simulink model "Ivanov_9_airplane"  (Simulink 10.0)
settings: Solver=FixedStepAuto  StartTime=0.0  StopTime=50.0  RelTol=1e-3
undefined symbols (not defined in the file or in its folder): DiscIntNeverNeededParam
libraries: aerolibanim x1
settings Model: Creator=prime  LastModifiedBy=prime
settings DataIOCC: SaveFormat=Dataset  ReturnWorkspaceOutputs=on
settings OptimizationCC: LifeSpan=auto
settings DebuggingCC: UnderspecifiedInitializationDetection=Simplified  MergeDetectMultiDrivingBlocksExec=error  SFUnexpectedBacktrackingDiag=error  SFNoUnconditionalDefaultTransitionDiag=error  SFExecutionAtInitializationDiag=warning  ArithmeticOperatorsInVariantConditions=error
settings HardwareCC: ProdBitPerPointer=64  ProdBitPerSizeT=64  ProdBitPerPtrDiffT=64  ProdLargestAtomicFloat=Float  ProdIntDivRoundTo=Zero  ProdEndianess=LittleEndian  ProdWordSize=64  ProdHWDeviceType=Intel->x86-64 (Windows64)
settings ModelReferenceCC: PropagateSignalLabelsOutOfModel=on
settings SFSimCC: SimUseLocalCustomCode=on  CustomCodeUndefinedFunction=FilterOut
settings RTWCC: RTWUseLocalCustomCode=on
settings CodeAppCC: StateflowObjectComments=off
settings GRTTargetCC: TargetLangStandard=C99 (ISO)  CombineOutputUpdateFcns=on  GRTInterface=off
settings ConfigComp: CovMetricSettings=dwe  CovHtmlReporting=off  CovSaveCumulativeToWorkspaceVar=off  CovSaveSingleToWorkspaceVar=off

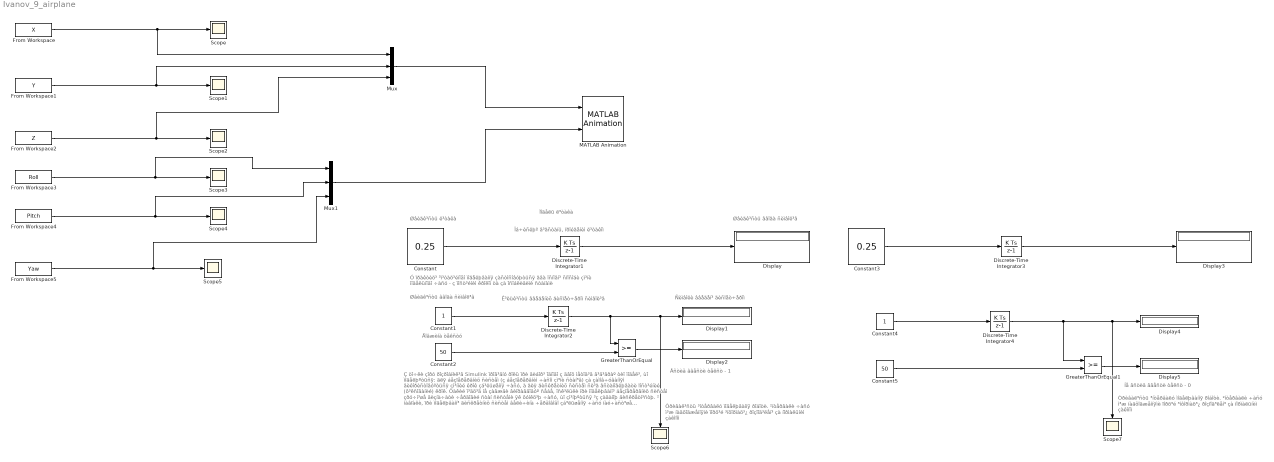
== system Ivanov_9_airplane ==
  note: Ñèìâîëè ââåäåí³ äèñïåò÷åðîì
  note: Øâèäê³ñòü ââîäà ñèìâîë³â
  note: Äîâæèíà òåêñòó
  note: Øâèäê³ñòü ë³òàêà
  note: Øâèäê³ñòü ââîäà ñèìâîë³â
  note: Âñòèã ââåñòè òåêñò - 1
  note: Îá÷èñëþº â³äñòàíü, ïðîéäåíèì ë³òàêîì
  note: Òðèâàë³ñòü ³íòåðâàëó ìîäåëþâàííÿ ðîáîòè.
      | ²íòåðâàëè ÷àñó ì³æ íàäõîäæåííÿìè ïîðö³é ³íôîðìàö³¿ ðîçïîä³ëåí³ çà íîðìàëüíèì çàêîíîì
  note: Íå âñòèã ââåñòè òåêñò - 0
  note: Òðèâàë³ñòü ³íòåðâàëó ìîäåëþâàííÿ ðîáîòè.
      | ²íòåðâàëè ÷àñó ì³æ íàäõîäæåííÿìè ïîðö³é ³íôîðìàö³¿ ðîçïîä³ëåí³ çà íîðìàëüíèì çàêîíîì
  note: Ê³ëüê³ñòü ââåäåíèõ äèñïåò÷åðîì ñèìâîë³â
  note: Ó ïðàêòèö³ ³ì³òàö³éíîãî ìîäåëþâàííÿ çàñòîñîâóþòüñÿ äâà îñíîâí³ ñïîñîáè çì³íè ìîäåëüíîãî ÷àñó - ç ïîñò³éíèì êðîêîì òà çà îñîáëèâèìè ñòàíàìè
  note: Ç òî÷êè çîðó ðîçðîáíèê³â Simulink ïðîâ³äíó ðîëü ïðè âèáîð³ îäíîãî ç äâîõ ìåòîä³â â³ä³ãðàº òèï ìîäåë³, ùî ìîäåëþºòüñÿ: äëÿ áåçïåðåðâíèõ ñèñòåì (ç áåçïåðåðâíèì ÷àñîì çì³íè ñòàí³â) çà çàìîâ÷óâàííÿì âèêîðèñòîâóºòüñÿ çì³ííèé êðîê çá³ëüøåííÿ ÷àñó, à äëÿ äèñêðåòíèõ ñèñòåì ñë³ä âñòàíîâëþâàòè ïîñò³éíèé (ô³êñîâàíèé) êðîê. Òàêèé ï³äõ³ä íå çàâæäè âèïðàâäîâóº ñåáå, îñê³ëüêè ïðè ìîäåëþâàíí³ áåçïåðåðâíèõ ñèñòåì çðó÷í³øå âèçíà÷àòè ÷åðãîâèé ñòàí ñèñòåìè ÿê ôóíêö³þ ÷àñó, ùî çì³íþºòüñÿ ³ç çàäàíîþ äèñêðåòí³ñòþ. ² íàâïàêè, ïðè ìîäåëþâàíí³ äèñêðåòíèõ ñèñòåì âåëè÷èíà ÷åðãîâîãî çá³ëüøåííÿ ÷àñó íàé÷àñò³øå âèçíà÷àºòüñÿ ïðîãíîçîâàíèì ìîìåíòîì çì³íè ñòàíó ñèñòåìè; ïðè÷îìó çì³íà ñòàí³â â³äáóâàºòüñÿ, çàçâè÷àé, íåðåãóëÿðíî. Òîìó êîðèñíî çíàòè, ÿêèì ÷èíîì ðîçðîáêè ìîäåëåé äèñêðåòíèõ ñèñòåì ìîæíà çìóñèòè ìîäåëüíèé ÷àñ çì³íþâàòèñÿ ïî îñîáëèâèì ñòàíàì.
  note: Ìîäåëü ë³òàêà
  Constant : Constant  Value=0.25  SampleTime=2
  Constant1 : Constant  SampleTime=2
  Constant2 : Constant  Value=50  SampleTime=2
  Constant3 : Constant  Value=0.25  SampleTime=3
  Constant4 : Constant  SampleTime=3
  Constant5 : Constant  Value=50  SampleTime=3
  Discrete-Time Integrator1 : DiscreteIntegrator  SampleTime=2  ICPrevOutput=DiscIntNeverNeededParam  ICPrevScaledInput=DiscIntNeverNeededParam
  Discrete-Time Integrator2 : DiscreteIntegrator  SampleTime=2  ICPrevOutput=DiscIntNeverNeededParam  ICPrevScaledInput=DiscIntNeverNeededParam
  Discrete-Time Integrator3 : DiscreteIntegrator  SampleTime=3  ICPrevOutput=DiscIntNeverNeededParam  ICPrevScaledInput=DiscIntNeverNeededParam
  Discrete-Time Integrator4 : DiscreteIntegrator  SampleTime=3  ICPrevOutput=DiscIntNeverNeededParam  ICPrevScaledInput=DiscIntNeverNeededParam
  Display{,1..5} (6 alike) : Display
      Display settings: Decimation=13
      Display1 settings: Decimation=50
      Display3 settings: Decimation=13
      Display4 settings: Decimation=50
  From Workspace : FromWorkspace  VariableName=X  SampleTime=2
  From Workspace1 : FromWorkspace  VariableName=Y  SampleTime=2
  From Workspace2 : FromWorkspace  VariableName=Z  SampleTime=2
  From Workspace3 : FromWorkspace  VariableName=Roll  SampleTime=2
  From Workspace4 : FromWorkspace  VariableName=Pitch  SampleTime=2
  From Workspace5 : FromWorkspace  VariableName=Yaw  SampleTime=2
  GreaterThanOrEqual : RelationalOperator  OutDataTypeStr=boolean  RndMeth=Simplest
  GreaterThanOrEqual1 : RelationalOperator  OutDataTypeStr=boolean  RndMeth=Simplest
  MATLAB Animation : aerolibanim/MATLAB Animation  Tag=Matlab Animation 6 DOF  Vehicles=1  Geometries='pa24-250_orange.ac'  BoundingBoxCoordinates=[-50,50,-50,50,-50,50]  CameraOffset=[-150,-50,0]  CameraViewAngle=3  SampleTime=0.01  FigurePosition=[1,49,1536,7.664000e+02]
      settings: SourceProductName=Aerospace Blockset  SourceProductBaseCode=AE
  Mux : Mux  Inputs=3
  Mux1 : Mux  Inputs=3
  Scope{,1..7} (8 alike) : Scope
  wires:
  From Workspace5/1 -> Mux1/3, Scope5/1
  From Workspace3/1 -> Mux1/1, Scope3/1
  From Workspace2/1 -> Mux/3, Scope2/1
  Mux1/1 -> MATLAB Animation/2
  From Workspace/1 -> Mux/1, Scope/1
  From Workspace4/1 -> Mux1/2, Scope4/1
  From Workspace1/1 -> Scope1/1, Mux/2
  Mux/1 -> MATLAB Animation/1
  Discrete-Time Integrator1/1 -> Display/1
  Constant/1 -> Discrete-Time Integrator1/1
  Constant1/1 -> Discrete-Time Integrator2/1
  Discrete-Time Integrator2/1 -> GreaterThanOrEqual/1, Scope6/1, Display1/1
  Constant2/1 -> GreaterThanOrEqual/2
  Constant5/1 -> GreaterThanOrEqual1/2
  GreaterThanOrEqual1/1 -> Display5/1
  Discrete-Time Integrator4/1 -> Scope7/1, Display4/1, GreaterThanOrEqual1/1
  Constant4/1 -> Discrete-Time Integrator4/1
  Constant3/1 -> Discrete-Time Integrator3/1
  Discrete-Time Integrator3/1 -> Display3/1
  GreaterThanOrEqual/1 -> Display2/1
